simulink model "DiscretePID"  (R2020b)
settings: Solver=FixedStepAuto  StartTime=0.0  StopTime=3  FixedStep=1e-4  RelTol=1e-4
undefined symbols (not defined in the file): daq, drv, gbox, mech, mld, mot, pid, rads2rpm, sens, sim
settings Model: Creator=Utente  LastModifiedBy=Utente

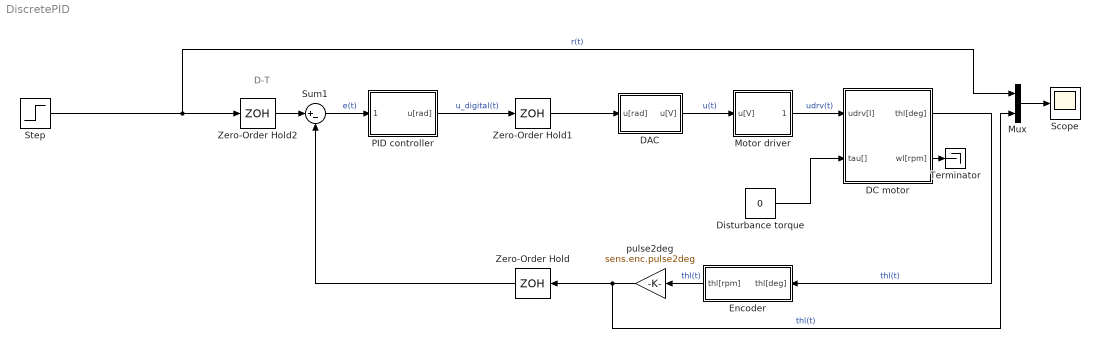
== system DiscretePID ==
  note: D-T
  DAC : Subsystem
  DC motor : Subsystem
  Disturbance torque : Constant  Value=0
  Encoder : Subsystem
  Motor driver : Subsystem
  Mux : Mux  Inputs=2
  PID controller : Subsystem
  Scope : Scope
  Step : Step  Time=0  After=50  SampleTime=0
  Sum1 : Sum  Inputs=|+-
  Terminator : Terminator
  Zero-Order Hold : ZeroOrderHold  SampleTime=sim.T_samp
  Zero-Order Hold1 : ZeroOrderHold  SampleTime=sim.T_samp
  Zero-Order Hold2 : ZeroOrderHold  SampleTime=sim.T_samp
  pulse2deg : Gain  Gain=sens.enc.pulse2deg
  wires:
  Disturbance torque/1 -> DC motor/2(tau[])
  Step/1 -> Mux/1, Zero-Order Hold2/1  "r(t)"
  Sum1/1 -> PID controller/1(e[deg])  "e(t)"
  DC motor/1(thl[deg]) -> Encoder/1(thl[deg])  "thl(t)"
  DAC/1(u[V]) -> Motor driver/1(u[V])  "u(t)"
  Mux/1 -> Scope/1
  pulse2deg/1 -> Mux/2, Zero-Order Hold/1  "thl(t)"
  Motor driver/1(udrv[I]) -> DC motor/1(udrv[I])  "udrv(t)"
  Encoder/1(thl[rpm]) -> pulse2deg/1  "thl(t)"
  Zero-Order Hold/1 -> Sum1/2
  PID controller/1(u[rad]) -> Zero-Order Hold1/1  "u_digital(t)"
  Zero-Order Hold1/1 -> DAC/1(u[rad])
  Zero-Order Hold2/1 -> Sum1/1
  DC motor/2(wl[rpm]) -> Terminator/1

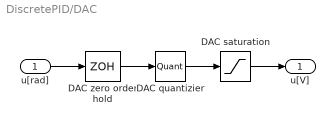
== system DiscretePID/DAC ==
  u[rad] : Inport
  DAC quantizier : Quantizer  QuantizationInterval=daq.dac.q
  DAC saturation : Saturate  UpperLimit=daq.dac.vdd  LowerLimit=daq.dac.vss
  DAC zero order hold : ZeroOrderHold  SampleTime=daq.dac.T_s
  u[V] : Outport
  wires:
  DAC quantizier/1 -> DAC saturation/1
  DAC zero order hold/1 -> DAC quantizier/1
  DAC saturation/1 -> u[V]/1
  u[rad]/1 -> DAC zero order hold/1

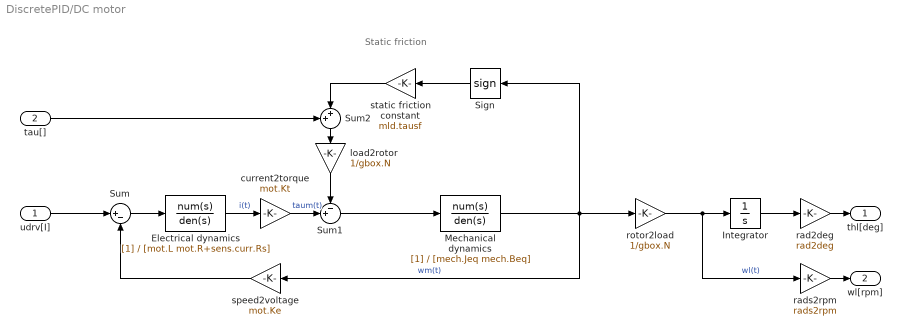
== system DiscretePID/DC motor ==
  note: Static friction
  udrv[I] : Inport  Unit=V
  tau[] : Inport  Port=2  Unit=V
  Electrical dynamics : TransferFcn  Denominator=[mot.L mot.R+sens.curr.Rs]
  Integrator : Integrator
  Mechanical dynamics : TransferFcn  Denominator=[mech.Jeq mech.Beq]
  Sign : Signum  ZeroCross=off
  Sum : Sum  Inputs=|+-
  Sum1 : Sum  Inputs=-+|
  Sum2 : Sum  Inputs=++|
  current2torque : Gain  Gain=mot.Kt
  load2rotor : Gain  Gain=1/gbox.N
  rad2deg : Gain  Gain=rad2deg
  rads2rpm : Gain  Gain=rads2rpm
  rotor2load : Gain  Gain=1/gbox.N
  speed2voltage : Gain  Gain=mot.Ke
  static friction constant : Gain  Gain=mld.tausf
  thl[deg] : Outport  Unit=deg
  wl[rpm] : Outport  Port=2  Unit=rpm
  wires:
  load2rotor/1 -> Sum1/1
  Mechanical dynamics/1 -> Sign/1, rotor2load/1, speed2voltage/1  "wm(t)"
  Sign/1 -> static friction constant/1
  current2torque/1 -> Sum1/2  "taum(t)"
  Sum1/1 -> Mechanical dynamics/1
  speed2voltage/1 -> Sum/2
  rotor2load/1 -> rads2rpm/1, Integrator/1  "wl(t)"
  Electrical dynamics/1 -> current2torque/1  "i(t)"
  Integrator/1 -> rad2deg/1
  Sum/1 -> Electrical dynamics/1
  rads2rpm/1 -> wl[rpm]/1
  rad2deg/1 -> thl[deg]/1
  udrv[I]/1 -> Sum/1
  static friction constant/1 -> Sum2/2
  Sum2/1 -> load2rotor/1
  tau[]/1 -> Sum2/1

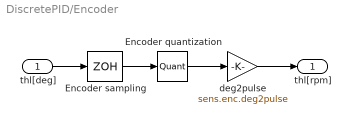
== system DiscretePID/Encoder ==
  thl[deg] : Inport
  Encoder quantization : Quantizer  QuantizationInterval=sens.enc.q
  Encoder sampling : ZeroOrderHold  SampleTime=sens.enc.T_s
  deg2pulse : Gain  Gain=sens.enc.deg2pulse
  thl[rpm] : Outport
  wires:
  Encoder quantization/1 -> deg2pulse/1
  deg2pulse/1 -> thl[rpm]/1
  Encoder sampling/1 -> Encoder quantization/1
  thl[deg]/1 -> Encoder sampling/1

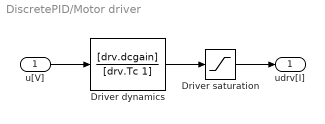
== system DiscretePID/Motor driver ==
  u[V] : Inport
  Driver dynamics : TransferFcn  Numerator=[drv.dcgain]  Denominator=[drv.Tc 1]
  Driver saturation : Saturate  UpperLimit=drv.vp  LowerLimit=drv.vm
  udrv[I] : Outport
  wires:
  Driver saturation/1 -> udrv[I]/1
  Driver dynamics/1 -> Driver saturation/1
  u[V]/1 -> Driver dynamics/1

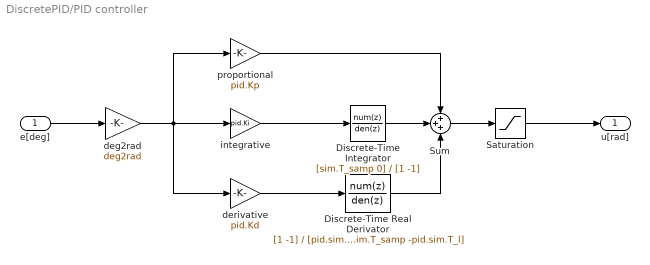
== system DiscretePID/PID controller ==
  e[deg] : Inport  Unit=deg
  Discrete-Time Integrator : DiscreteTransferFcn  Numerator=[sim.T_samp 0]  Denominator=[1 -1]  SampleTime=sim.T_samp
  Discrete-Time Real Derivator : DiscreteTransferFcn  Numerator=[1 -1]  Denominator=[pid.sim.T_l+sim.T_samp -pid.sim.T_l]  SampleTime=sim.T_samp
  Saturation : Saturate  UpperLimit=daq.dac.vdd  LowerLimit=daq.dac.vss
  Sum : Sum  Inputs=+++
  deg2rad : Gain  Gain=deg2rad
  derivative : Gain  Gain=pid.Kd
  integrative : Gain  Gain=pid.Ki
  proportional : Gain  Gain=pid.Kp
  u[rad] : Outport
  wires:
  e[deg]/1 -> deg2rad/1
  Sum/1 -> Saturation/1
  deg2rad/1 -> proportional/1, integrative/1, derivative/1
  proportional/1 -> Sum/1
  integrative/1 -> Discrete-Time Integrator/1
  Saturation/1 -> u[rad]/1
  derivative/1 -> Discrete-Time Real Derivator/1
  Discrete-Time Integrator/1 -> Sum/2
  Discrete-Time Real Derivator/1 -> Sum/3
